simulink model "autopilot_deneme"  (R2020b)
settings: Solver=VariableStepAuto  StartTime=0.0  StopTime=300  RelTol=1e-3
values from neighbouring files (symbols this model uses):
  u1max = 25*pi/180    (= 0.436332312999)    [RCAM_initialization.m]
  u1min = -25*pi/180    (= -0.436332312999)    [RCAM_initialization.m]
  u2max = 10*pi/180    (= 0.174532925199)    [RCAM_initialization.m]
  u2min = -25*pi/180    (= -0.436332312999)    [RCAM_initialization.m]
  u3max = 30*pi/180    (= 0.523598775598)    [RCAM_initialization.m]
  u3min = -30*pi/180    (= -0.523598775598)    [RCAM_initialization.m]
  u4max = 10*pi/180    (= 0.174532925199)    [RCAM_initialization.m]
  u4min = 0.5*pi/180    (= 0.00872664625997)    [RCAM_initialization.m]
  u5max = 10*pi/180    (= 0.174532925199)    [RCAM_initialization.m]
  u5min = 0.5*pi/180    (= 0.00872664625997)    [RCAM_initialization.m]
  x0 = [85; 0; 0; 0; 0; 0; 0; 0; 0; xini; yini; h0]    [RCAM_initialization.m]
undefined symbols (not defined in the file or in its folder): RCAM_MODEL
libraries: aerolibfltsims x2, AE512Blockset x2, pid_lib x2, aerolibatmos2 x1
settings Model: Creator=Yigit  LastModifiedBy=Yigit

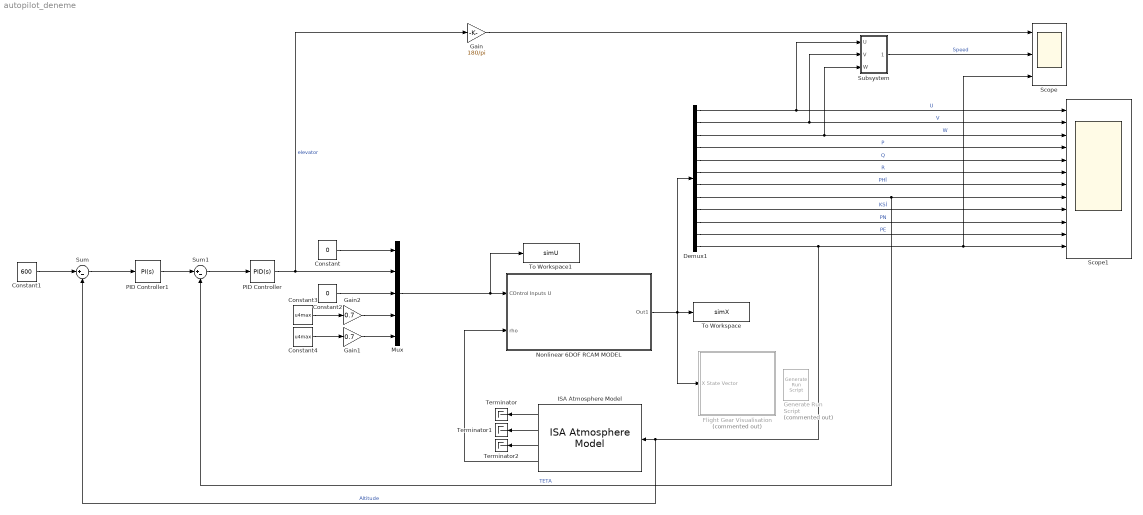
== system autopilot_deneme ==
  Constant : Constant  Value=0
  Constant1 : Constant  Value=600
  Constant2 : Constant  Value=0
  Constant3 : Constant  Value=u4max
  Constant4 : Constant  Value=u4max
  Demux1 : Demux  Outputs=12
  Flight Gear Visualisation : Subsystem  Commented=on
  Gain : Gain  Gain=180/pi
  Gain1 : Gain  Gain=0.7
  Gain2 : Gain  Gain=0.7
  Generate Run Script : aerolibfltsims/Generate Run Script  Commented=on  Architecture=Default  dataFlow=Send  GeometryModelName=737-300  AirportId=KSFO  RunwayId=10L  InitialAltitude=7224  InitialHeading=113  OffsetDistance=4.72  OffsetAzimuth=0  InstallScenery=off  DisableShaders=on  OriginAddress=127.0.0.1  DestinationPort=5502  OriginPort=5505  LocalAddress=127.0.0.1  OutputFileName=runfg.bat  FlightGearBaseDirectory=C:\Program Files\FlightGear 2020.3
  ISA Atmosphere Model : aerolibatmos2/ISA Atmosphere Model  custom=off  g=9.80665  gamma=1.4  R=287.0531  L=0.0065  h_trop=11000  h_strat=20000  rho0=1.225  P0=101325  T0=288.15  h0=0
  Mux : Mux  Inputs=5
  Nonlinear 6DOF RCAM MODEL : Subsystem
      mask Display: image('C:\Users\Yigit\Downloads\plane.png'); % Use "Edit Image" on toolstrip to change.
  PID Controller : pid_lib/PID Controller  Controller=PID  Form=Parallel  TimeDomain=Continuous-time  UseExternalTs=off  SampleTime=-1  IntegratorMethod=Forward Euler  FilterMethod=Forward Euler  ControllerParametersSource=internal  P=-10.4422065862057  I=-5.87025518887093  D=-4.60177988709861  UseFilter=on  N=1482.11840390405  TunerSelectOption=Transfer Function Based (PID Tuner App)  InitialConditionSource=internal  InitialConditionForIntegrator=0  InitialConditionForFilter=0  DifferentiatorICPrevScaledInput=0  ExternalReset=none  TrackingMode=off  Kt=1  LimitOutput=on  SatLimitsSource=internal  UpperSaturationLimit=u2max  LowerSaturationLimit=u2min  LinearizeAsGain=on  AntiWindupMode=back-calculation  Kb=1  POutMin=[]  POutMax=[]  IOutMin=[]  IOutMax=[]  DOutMin=[]  DOutMax=[]  NOutMin=[]  NOutMax=[]  SumOutMin=[]  SumOutMax=[]  SaturationOutMin=[]  SaturationOutMax=[]  PParamMin=[]  PParamMax=[]  IParamMin=[]  IParamMax=[]  DParamMin=[]  DParamMax=[]  NParamMin=[]  NParamMax=[]  KbParamMin=[]  KbParamMax=[]  KtParamMin=[]  KtParamMax=[]  KbOutMin=[]  KbOutMax=[]  KtOutMin=[]  KtOutMax=[]  IntegratorOutMin=[]  IntegratorOutMax=[]  FilterOutMin=[]  FilterOutMax=[]  SumI1OutMin=[]  SumI1OutMax=[]  SumI2OutMin=[]  SumI2OutMax=[]  SumI3OutMin=[]  SumI3OutMax=[]  SumI4OutMin=[]  SumI4OutMax=[]  SumDOutMin=[]  SumDOutMax=[]  DifferentiatorOutMin=[]  DifferentiatorOutMax=[]  FilterDiffOutCoefMin=[]  FilterDiffOutCoefMax=[]  ReciprocalOutMin=[]  ReciprocalOutMax=[]  SumDenOutMin=[]  SumDenOutMax=[]  SumNumOutMin=[]  SumNumOutMax=[]  DivideOutMin=[]  DivideOutMax=[]  UdiffTsProdOutMin=[]  UdiffTsProdOutMax=[]  NTsProdOutMin=[]  NTsProdOutMax=[]  UintegralTsProdOutMin=[]  UintegralTsProdOutMax=[]  UngainTsProdOutMin=[]  UngainTsProdOutMax=[]  IntegratorContinuousStateAttributes=''  IntegratorStateMustResolveToSignalObject=off  IntegratorRTWStateStorageClass=Auto  FilterContinuousStateAttributes=''  FilterStateMustResolveToSignalObject=off  FilterRTWStateStorageClass=Auto  ParallelPVariant=InternalParameters  IdealPVariant=Disabled  IVariant=InternalParameters  DVariant=InternalParameters  IntegratorVariant=Continuous  SatVariant=Enabled  AWVariant=BackCalculation  PCopyVariant=Disabled  TRVariant=Disabled  FdbkBlocksVariant=Forward  IdealPFdbkVariant=Disabled  SatFdbkVariant=Disabled  DerivativeFilterVariant=ContFilter  NVariant=InternalParameters  NCopyVariant=Disabled  FilterICVariant=InternalICsFilter  IntegratorICVariant=InternalICs  ExternalResetVariant=Disabled  TRSumVariant=Passthrough  SumFdbkVariant=Disabled  SumVariant=Sum_PID  TsampFilterVariant=InternalTs  TsampNgainVariant=Passthrough  TsampIntegralVariant=Passthrough  ExternalSaturationOutDataTypeStr=Inherit: Same as second input
  PID Controller1 : pid_lib/PID Controller  Controller=PI  Form=Parallel  TimeDomain=Continuous-time  UseExternalTs=off  SampleTime=-1  IntegratorMethod=Forward Euler  FilterMethod=Forward Euler  ControllerParametersSource=internal  P=0.00272431164108648  I=0.00012875407275399  D=0.00175748492645377  UseFilter=on  N=7.36999853508895  TunerSelectOption=Transfer Function Based (PID Tuner App)  InitialConditionSource=internal  InitialConditionForIntegrator=0  InitialConditionForFilter=0  DifferentiatorICPrevScaledInput=0  ExternalReset=none  TrackingMode=off  Kt=1  LimitOutput=off  SatLimitsSource=internal  UpperSaturationLimit=u2max  LowerSaturationLimit=u2min  LinearizeAsGain=on  AntiWindupMode=none  Kb=1  POutMin=[]  POutMax=[]  IOutMin=[]  IOutMax=[]  DOutMin=[]  DOutMax=[]  NOutMin=[]  NOutMax=[]  SumOutMin=[]  SumOutMax=[]  SaturationOutMin=[]  SaturationOutMax=[]  PParamMin=[]  PParamMax=[]  IParamMin=[]  IParamMax=[]  DParamMin=[]  DParamMax=[]  NParamMin=[]  NParamMax=[]  KbParamMin=[]  KbParamMax=[]  KtParamMin=[]  KtParamMax=[]  KbOutMin=[]  KbOutMax=[]  KtOutMin=[]  KtOutMax=[]  IntegratorOutMin=[]  IntegratorOutMax=[]  FilterOutMin=[]  FilterOutMax=[]  SumI1OutMin=[]  SumI1OutMax=[]  SumI2OutMin=[]  SumI2OutMax=[]  SumI3OutMin=[]  SumI3OutMax=[]  SumI4OutMin=[]  SumI4OutMax=[]  SumDOutMin=[]  SumDOutMax=[]  DifferentiatorOutMin=[]  DifferentiatorOutMax=[]  FilterDiffOutCoefMin=[]  FilterDiffOutCoefMax=[]  ReciprocalOutMin=[]  ReciprocalOutMax=[]  SumDenOutMin=[]  SumDenOutMax=[]  SumNumOutMin=[]  SumNumOutMax=[]  DivideOutMin=[]  DivideOutMax=[]  UdiffTsProdOutMin=[]  UdiffTsProdOutMax=[]  NTsProdOutMin=[]  NTsProdOutMax=[]  UintegralTsProdOutMin=[]  UintegralTsProdOutMax=[]  UngainTsProdOutMin=[]  UngainTsProdOutMax=[]  IntegratorContinuousStateAttributes=''  IntegratorStateMustResolveToSignalObject=off  IntegratorRTWStateStorageClass=Auto  FilterContinuousStateAttributes=''  FilterStateMustResolveToSignalObject=off  FilterRTWStateStorageClass=Auto  ParallelPVariant=InternalParameters  IdealPVariant=Disabled  IVariant=InternalParameters  DVariant=Disabled  IntegratorVariant=Continuous  SatVariant=Disabled  AWVariant=Passthrough  PCopyVariant=Disabled  TRVariant=Disabled  FdbkBlocksVariant=Forward  IdealPFdbkVariant=Disabled  SatFdbkVariant=Disabled  DerivativeFilterVariant=Disabled  NVariant=Disabled  NCopyVariant=Disabled_SignalSpec  FilterICVariant=Disabled  IntegratorICVariant=InternalICs  ExternalResetVariant=Disabled  TRSumVariant=Passthrough  SumFdbkVariant=Disabled  SumVariant=Sum_PI  TsampFilterVariant=InternalTs  TsampNgainVariant=Passthrough  TsampIntegralVariant=Passthrough  ExternalSaturationOutDataTypeStr=Inherit: Same as second input
  Scope : Scope  NumInputPorts=3
  Scope1 : Scope  NumInputPorts=12
  Subsystem : Subsystem
  Sum : Sum  Inputs=|+-
  Sum1 : Sum  Inputs=|+-
  Terminator : Terminator
  Terminator1 : Terminator
  Terminator2 : Terminator
  To Workspace : ToWorkspace  VariableName=simX  SaveFormat=Timeseries  SampleTime=-1
  To Workspace1 : ToWorkspace  VariableName=simU  SaveFormat=Timeseries  SampleTime=-1
  wires:
  Nonlinear 6DOF RCAM MODEL/1(Out1) -> Flight Gear Visualisation/1(X State Vector), Demux1/1, To Workspace/1
  ISA Atmosphere Model/2 -> Terminator1/1
  ISA Atmosphere Model/3 -> Terminator2/1
  Demux1/3 -> Scope1/3, Subsystem/3(W)  "W"
  Demux1/2 -> Scope1/2, Subsystem/2(V)  "V"
  Demux1/5 -> Scope1/5  "Q"
  Demux1/12 -> ISA Atmosphere Model/1, Sum/2, Scope/3, Scope1/12  "Altitude"
  ISA Atmosphere Model/1 -> Terminator/1
  Demux1/10 -> Scope1/10  "PN"
  Demux1/7 -> Scope1/7  "PHİ"
  ISA Atmosphere Model/4 -> Nonlinear 6DOF RCAM MODEL/2(rho)
  Demux1/11 -> Scope1/11  "PE"
  Demux1/8 -> Scope1/8, Sum1/2  "TETA"
  Demux1/9 -> Scope1/9  "KSİ"
  Demux1/1 -> Subsystem/1(U), Scope1/1  "U"
  Demux1/6 -> Scope1/6  "R"
  Mux/1 -> To Workspace1/1, Nonlinear 6DOF RCAM MODEL/1(COntrol Inputs U)
  Demux1/4 -> Scope1/4  "P"
  Constant1/1 -> Sum/1
  Constant/1 -> Mux/1
  Constant2/1 -> Mux/3
  Constant3/1 -> Gain2/1
  Constant4/1 -> Gain1/1
  PID Controller/1 -> Gain/1, Mux/2  "elevator"
  Subsystem/1(Out1) -> Scope/2  "Speed"
  Gain/1 -> Scope/1
  Sum/1 -> PID Controller1/1
  PID Controller1/1 -> Sum1/1
  Sum1/1 -> PID Controller/1
  Gain1/1 -> Mux/5
  Gain2/1 -> Mux/4

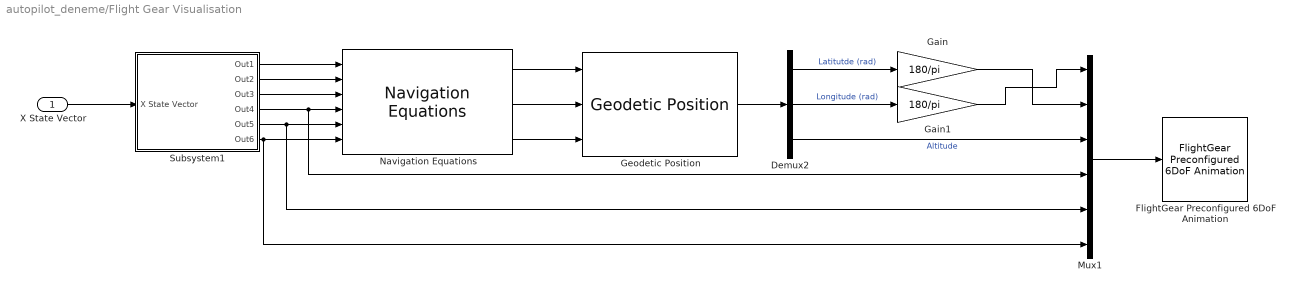
== system autopilot_deneme/Flight Gear Visualisation ==
  X State Vector : Inport
  Demux2 : Demux  Outputs=3
  FlightGear Preconfigured 6DoF Animation : aerolibfltsims/FlightGear Preconfigured 6DoF Animation  xFlightGearVersion=v2019.1  DestinationIpAddress=127.0.0.1  DestinationPort=5502  SampleTime=1/30  packetVersion=24
  Gain : Gain  Gain=180/pi
  Gain1 : Gain  Gain=180/pi
  Geodetic Position : AE512Blockset/Geodetic Position  Xgeodetic0=Xgeodetic0
  Mux1 : Mux  Inputs=6
  Navigation Equations : AE512Blockset/Navigation Equations  Description=|
      | Version History  
      |                  
      | 05/24/05: Created
  Subsystem1 : Subsystem
  wires:
  Subsystem1/2(Out2) -> Navigation Equations/2
  Subsystem1/6(Out6) -> Mux1/6, Navigation Equations/6
  Demux2/2 -> Gain1/1  "Longitude (rad)"
  Subsystem1/1(Out1) -> Navigation Equations/1
  Geodetic Position/1 -> Demux2/1
  Gain/1 -> Mux1/2
  Subsystem1/4(Out4) -> Mux1/4, Navigation Equations/4
  Demux2/1 -> Gain/1  "Latitutde (rad)"
  Subsystem1/3(Out3) -> Navigation Equations/3
  Mux1/1 -> FlightGear Preconfigured 6DoF Animation/1
  Demux2/3 -> Mux1/3  "Altitude"
  Gain1/1 -> Mux1/1
  Subsystem1/5(Out5) -> Mux1/5, Navigation Equations/5
  Navigation Equations/1 -> Geodetic Position/1
  Navigation Equations/3 -> Geodetic Position/3
  Navigation Equations/2 -> Geodetic Position/2
  X State Vector/1 -> Subsystem1/1(X State Vector)

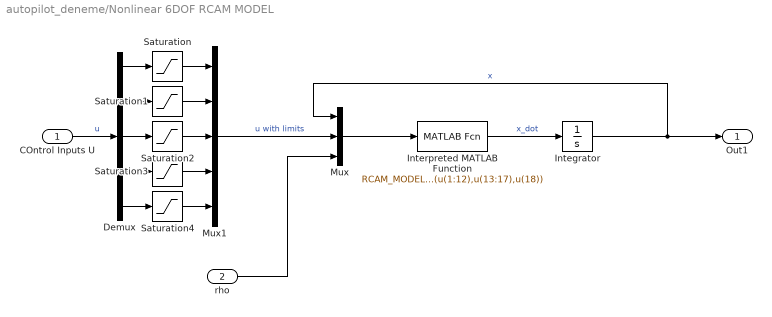
== system autopilot_deneme/Nonlinear 6DOF RCAM MODEL ==
  COntrol Inputs U : Inport
  rho : Inport  Port=2
  Demux : Demux  Outputs=5
  Integrator : Integrator  InitialCondition=x0
  Interpreted MATLAB Function : MATLABFcn  MATLABFcn=RCAM_MODEL(u(1:12),u(13:17),u(18))
  Mux : Mux  Inputs=3
  Mux1 : Mux  Inputs=5
  Saturation : Saturate  UpperLimit=u1max  LowerLimit=u1min
  Saturation1 : Saturate  UpperLimit=u2max  LowerLimit=u2min
  Saturation2 : Saturate  UpperLimit=u3max  LowerLimit=u3min
  Saturation3 : Saturate  UpperLimit=u4max  LowerLimit=u4min
  Saturation4 : Saturate  UpperLimit=u5max  LowerLimit=u5min
  Out1 : Outport
  wires:
  Interpreted MATLAB Function/1 -> Integrator/1  "x_dot"
  Mux/1 -> Interpreted MATLAB Function/1
  Integrator/1 -> Out1/1, Mux/1  "x"
  COntrol Inputs U/1 -> Demux/1  "u"
  Demux/1 -> Saturation/1
  Demux/4 -> Saturation3/1
  Demux/5 -> Saturation4/1
  Demux/3 -> Saturation2/1
  Demux/2 -> Saturation1/1
  Saturation3/1 -> Mux1/4
  Saturation4/1 -> Mux1/5
  Saturation2/1 -> Mux1/3
  Saturation1/1 -> Mux1/2
  Saturation/1 -> Mux1/1
  Mux1/1 -> Mux/2  "u with limits"
  rho/1 -> Mux/3

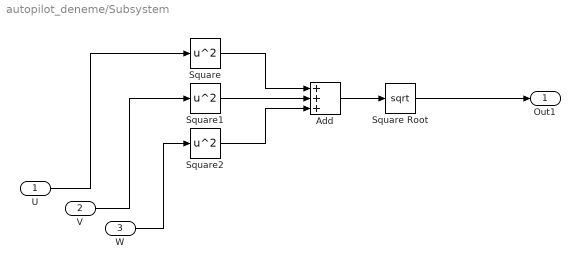
== system autopilot_deneme/Subsystem ==
  U : Inport
  V : Inport  Port=2
  W : Inport  Port=3
  Add : Sum  Inputs=+++
  Square : Math  Operator=square  SaturateOnIntegerOverflow=on
  Square Root : Sqrt  SaturateOnIntegerOverflow=on
  Square1 : Math  Operator=square  SaturateOnIntegerOverflow=on
  Square2 : Math  Operator=square  SaturateOnIntegerOverflow=on
  Out1 : Outport
  wires:
  V/1 -> Square1/1
  Add/1 -> Square Root/1
  Square2/1 -> Add/3
  Square Root/1 -> Out1/1
  Square1/1 -> Add/2
  W/1 -> Square2/1
  Square/1 -> Add/1
  U/1 -> Square/1

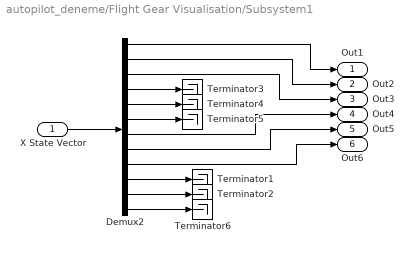
== system autopilot_deneme/Flight Gear Visualisation/Subsystem1 ==
  X State Vector : Inport
  Demux2 : Demux  Outputs=12
  Terminator{1..6} (6 alike) : Terminator
  Out1 : Outport
  Out2 : Outport  Port=2
  Out3 : Outport  Port=3
  Out4 : Outport  Port=4
  Out5 : Outport  Port=5
  Out6 : Outport  Port=6
  wires:
  Demux2/3 -> Out3/1
  X State Vector/1 -> Demux2/1
  Demux2/5 -> Terminator4/1
  Demux2/7 -> Out4/1
  Demux2/4 -> Terminator3/1
  Demux2/1 -> Out1/1
  Demux2/6 -> Terminator5/1
  Demux2/9 -> Out6/1
  Demux2/2 -> Out2/1
  Demux2/8 -> Out5/1
  Demux2/10 -> Terminator1/1
  Demux2/11 -> Terminator2/1
  Demux2/12 -> Terminator6/1
